simulink model "ofb2"  (R2016b)
settings: Solver=VariableStepAuto  StartTime=0.0  StopTime=tfinal  RelTol=1e-3  EnableMultiTasking=on
values from neighbouring files (symbols this model uses):
  Ts_fofb = 10e-6    (= 1e-05)    [simofbsirius.m]
  Ts_sofb = 1e-3    (= 0.001)    [simofbsirius.m]
libraries: cstblocks x5
settings Model: Creator=daniel.tavares  LastModifiedBy=danielot
settings DataIOCC: ExternalInput=simsignals  LoadExternalInput=on  SaveFormat=StructureWithTime  SignalLoggingSaveFormat=ModelDataLogs  SignalLogging=off  DSMLogging=off
settings OptimizationCC: ExpressionDepthLimit=2147483647  LifeSpan=inf
settings DebuggingCC: AlgebraicLoopMsg=none  ArtificialAlgebraicLoopMsg=none  UnderspecifiedInitializationDetection=Classic  MergeDetectMultiDrivingBlocksExec=none  SolverPrmCheckMsg=warning  FcnCallInpInsideContextMsg=warning  ModelReferenceExtraNoncontSigs=none  StateNameClashWarn=warning  SFUnexpectedBacktrackingDiag=warning  SFNoUnconditionalDefaultTransitionDiag=warning  SFExecutionAtInitializationDiag=none
settings HardwareCC: ProdBitPerPointer=32  ProdBitPerSizeT=32  ProdBitPerPtrDiffT=32  ProdLargestAtomicFloat=None  ProdIntDivRoundTo=Undefined  ProdEndianess=Unspecified  ProdWordSize=32  ProdHWDeviceType=32-bit Generic
settings ModelReferenceCC: PropagateSignalLabelsOutOfModel=off
settings GRTTargetCC: TargetLangStandard=C89/C90 (ANSI)  GeneratePreprocessorConditionals=Disable all  CombineOutputUpdateFcns=off  GRTInterface=on
settings ConfigComp: CovMetricSettings=dw  CovHtmlReporting=on  CovSaveCumulativeToWorkspaceVar=on  CovSaveSingleToWorkspaceVar=on  CovExternalEMLEnable=off

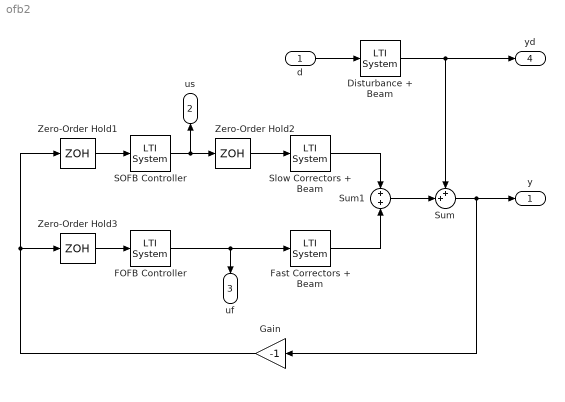
== system ofb2 ==
  d : Inport  PortDimensions=ndist  SampleTime=Ts_fofb
  Disturbance + Beam : cstblocks/LTI System  sys=D  IC=[]
  FOFB Controller : cstblocks/LTI System  sys=Cf  IC=[]
  Fast Correctors + Beam : cstblocks/LTI System  sys=Pf  IC=[]
  Gain : Gain  Gain=-1
  SOFB Controller : cstblocks/LTI System  sys=Cs  IC=[]
  Slow Correctors + Beam : cstblocks/LTI System  sys=Ps  IC=[]
  Sum : Sum  Inputs=++|
  Sum1 : Sum  Inputs=+|+
  Zero-Order Hold1 : ZeroOrderHold  SampleTime=Ts_sofb
  Zero-Order Hold2 : ZeroOrderHold  SampleTime=Ts_fofb
  Zero-Order Hold3 : ZeroOrderHold  SampleTime=Ts_fofb
  y : Outport
  us : Outport  Port=2
  uf : Outport  Port=3
  yd : Outport  Port=4
  wires:
  Sum/1 -> y/1, Gain/1
  FOFB Controller/1 -> Fast Correctors + Beam/1, uf/1
  SOFB Controller/1 -> us/1, Zero-Order Hold2/1
  Zero-Order Hold2/1 -> Slow Correctors + Beam/1
  Zero-Order Hold1/1 -> SOFB Controller/1
  Zero-Order Hold3/1 -> FOFB Controller/1
  d/1 -> Disturbance + Beam/1
  Disturbance + Beam/1 -> yd/1, Sum/1
  Sum1/1 -> Sum/2
  Slow Correctors + Beam/1 -> Sum1/1
  Fast Correctors + Beam/1 -> Sum1/2
  Gain/1 -> Zero-Order Hold3/1, Zero-Order Hold1/1
